simulink model "Full_cubesat"  (Simulink 7.9)
settings: Solver=ode45  StartTime=0.0  StopTime=10.0  RelTol=1e-3
values from neighbouring files (symbols this model uses):
  A_attitude_dynamics = [ 0 0 0 I1/Ix 0 0 ... (first row only)    [MatrixSetup.m]
  B_attitude_dynamics = [0 0 0 0 0 0 ... (first row only)    [MatrixSetup.m]
  C_attitude_dynamics = eye(6)    [MatrixSetup.m]
  D_attitude_dynamics = zeros(6)    [MatrixSetup.m]
settings Model: Creator=Dmitriy  LastModifiedBy=Dmitriy

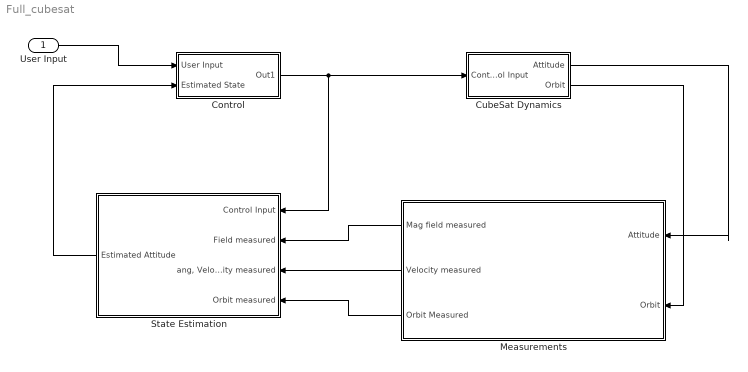
== system Full_cubesat ==
  User Input : Inport
  Control : Subsystem
  CubeSat Dynamics : Subsystem
  Measurements : Subsystem
  State Estimation : Subsystem
  wires:
  User Input/1 -> Control/1(User Input)
  State Estimation/1(Estimated Attitude) -> Control/2(Estimated State)
  Control/1(Out1) -> CubeSat Dynamics/1(Control Input), State Estimation/1(Control Input)
  CubeSat Dynamics/1(Attitude) -> Measurements/1(Attitude)
  CubeSat Dynamics/2(Orbit) -> Measurements/2(Orbit)
  Measurements/1(Mag field measured) -> State Estimation/2(Field measured)
  Measurements/2(Velocity measured) -> State Estimation/3("ang, Velocity measured")
  Measurements/3(Orbit Measured) -> State Estimation/4(Orbit measured)

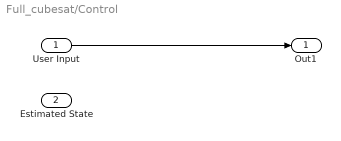
== system Full_cubesat/Control ==
  User Input : Inport
  Estimated State : Inport  Port=2
  Out1 : Outport
  wires:
  User Input/1 -> Out1/1

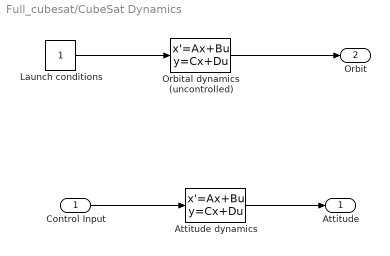
== system Full_cubesat/CubeSat Dynamics ==
  Control Input : Inport
  Attitude dynamics : StateSpace  A=A_attitude_dynamics  B=B_attitude_dynamics  C=C_attitude_dynamics  D=D_attitude_dynamics
  Launch conditions : Constant
  Orbital dynamics (uncontrolled) : StateSpace
  Attitude : Outport
  Orbit : Outport  Port=2
  wires:
  Control Input/1 -> Attitude dynamics/1
  Attitude dynamics/1 -> Attitude/1
  Launch conditions/1 -> Orbital dynamics (uncontrolled)/1
  Orbital dynamics (uncontrolled)/1 -> Orbit/1

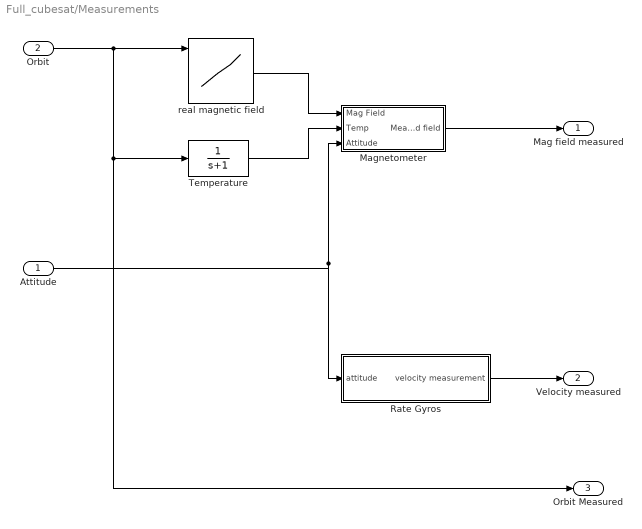
== system Full_cubesat/Measurements ==
  Attitude : Inport
  Orbit : Inport  Port=2
  Magnetometer : Subsystem
  Rate Gyros : Subsystem
  Temperature : TransferFcn  Denominator=[1 1]
  real magnetic field : Lookup_n-D  NumberOfTableDimensions=4  BreakpointsForDimension3=[5, 7]  Table=reshape(repmat([4 5 6;16 19 20;10 18 23],1,2),[3,3,2])  RndMeth=Simplest  InputSameDT=on
  Mag field measured : Outport
  Velocity measured : Outport  Port=2
  Orbit Measured : Outport  Port=3
  wires:
  Orbit/1 -> real magnetic field/1, Temperature/1, Orbit Measured/1
  real magnetic field/1 -> Magnetometer/1(Mag Field)
  Temperature/1 -> Magnetometer/2(Temp)
  Magnetometer/1(Measured field) -> Mag field measured/1
  Attitude/1 -> Magnetometer/3(Attitude), Rate Gyros/1(attitude)
  Rate Gyros/1(velocity measurement) -> Velocity measured/1

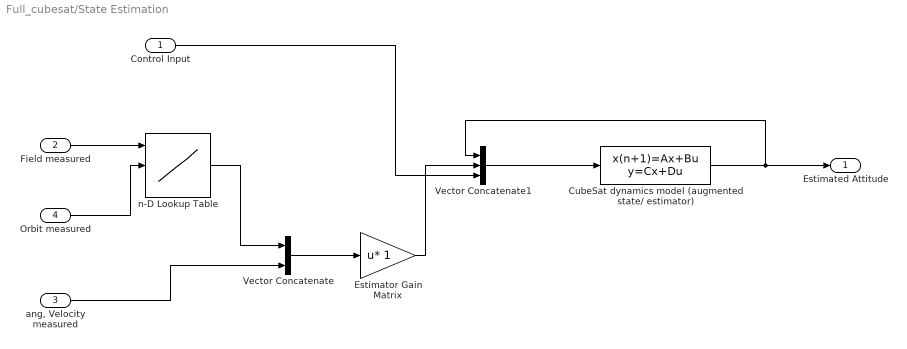
== system Full_cubesat/State Estimation ==
  Control Input : Inport
  Field measured : Inport  Port=2
  "ang, Velocity measured" : Inport  Port=3
  Orbit measured : Inport  Port=4
  CubeSat dynamics model (augmented state/ estimator) : DiscreteStateSpace
  Estimator Gain Matrix : Gain  Multiplication=Matrix(u*K)
  Vector Concatenate : Concatenate
  Vector Concatenate1 : Concatenate  NumInputs=3
  n-D Lookup Table : Lookup_n-D  NumberOfTableDimensions=3  BreakpointsForDimension3=[5, 7]  Table=reshape(repmat([4 5 6;16 19 20;10 18 23],1,2),[3,3,2])  RndMeth=Simplest  InputSameDT=on
  Estimated Attitude : Outport
  wires:
  Field measured/1 -> n-D Lookup Table/1
  Orbit measured/1 -> n-D Lookup Table/2
  CubeSat dynamics model (augmented state/ estimator)/1 -> Estimated Attitude/1, Vector Concatenate1/1
  n-D Lookup Table/1 -> Vector Concatenate/1
  "ang, Velocity measured"/1 -> Vector Concatenate/2
  Vector Concatenate/1 -> Estimator Gain Matrix/1
  Vector Concatenate1/1 -> CubeSat dynamics model (augmented state/ estimator)/1
  Estimator Gain Matrix/1 -> Vector Concatenate1/2
  Control Input/1 -> Vector Concatenate1/3

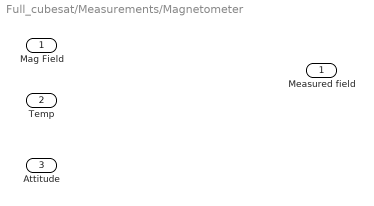
== system Full_cubesat/Measurements/Magnetometer ==
  Mag Field : Inport
  Temp : Inport  Port=2
  Attitude : Inport  Port=3
  Measured field : Outport

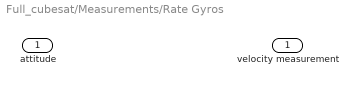
== system Full_cubesat/Measurements/Rate Gyros ==
  attitude : Inport
  velocity measurement : Outport
